simulink library "PEACDC01MSEREF"  (R2014b)
settings: Solver=ode45  StartTime=0.0  StopTime=10.0  RelTol=1e-3
undefined symbols (not defined in the file): errordlg
libraries: simulink x6
settings Model: Creator=vda2sh  LastModifiedBy=vda2sh
settings OptimizationCC: UseDivisionForNetSlopeComputation=off  SimCompilerOptimization=off
settings DebuggingCC: FrameProcessingCompatibilityMsg=error  AllowSymbolicDim=off
settings RTWCC: RTWCompilerOptimization=off
settings ConfigComp: CovMetricSettings=dw  CovHtmlReporting=on  CovSaveCumulativeToWorkspaceVar=on  CovSaveSingleToWorkspaceVar=on  CovModelRefEnable=Off  CovExternalEMLEnable=off  CovSFcnEnable=off

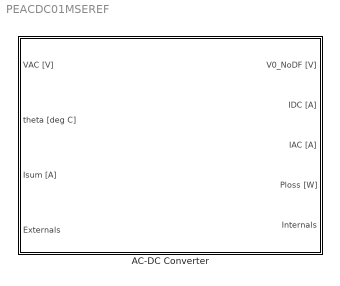
== system PEACDC01MSEREF ==
  "AC-DC Converter " : Subsystem  Tag=PEACDC01MSEREF  RequirementInfo="{}  %GIDa_5dfe5db4_0575_4ff1_ab59_fb674d557647"  mask(PEACDC01MSEREF){VD20=0.7, RD20=1e-3, alphaVD=0.0, alphaRD=0.0}
      mask prompts: VD20 "Diode forward voltage at 20°C [V]"; RD20 "Diode on resistance at 20°C [Ohm]"; alphaVD "Thermal coefficient of diode forward voltage [1/K]"; alphaRD "Thermal coefficient of diode on resistance [1/K]"
      mask help:
      | PEACDC01MSEREF - AC-DC converter
      |
      | This is a model of an AC-DC converter. It represents a full-wave rectifier using 4 diodes.
      settings: AttributesFormatString=<%<Tag>>
      mask Help: eval('show_docs_mseref_powerelectronics(''PEACDC01MSEREF'')')
      mask Display:
      | image(imread('PEACDC01MSEREF.jpg'),[0.16, 0.15, 0.73, 0.7]);
      | port_label('input',1,'VAC [V]')
      | port_label('input',2,'theta [°C]')
      | port_label('input',3,'Isum [A]')
      | port_label('input',4,'Externals')
      | port_label('output',1,'V0_NoDF [V]')
      | port_label('output',2,'IDC [A]')
      | port_label('output',3,'IAC [A]')
      | port_label('output',4,'Ploss [W]')
      | port_label('output',5,'Internals')

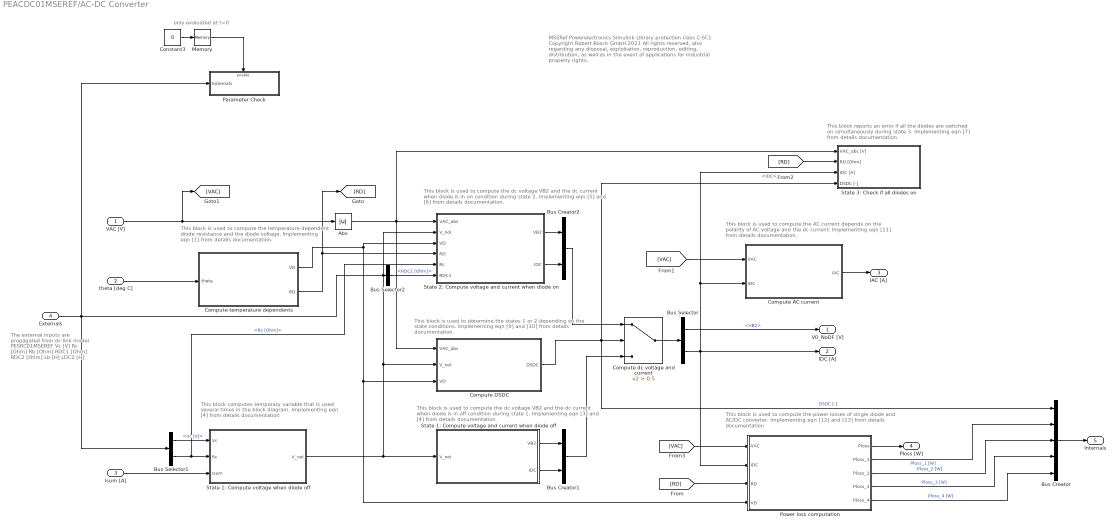
== system PEACDC01MSEREF/AC-DC Converter  ==
  note: The external inputs are
      | propagated from dc-link
      | model PESRC01MSEREF
      |
      | Vc [V]
      | Rc [Ohm]
      | Rb [Ohm]
      | RDC1 [Ohm]
      | RDC2 [Ohm]
      | Lb [H]
      | LDC2 [H]
  note: This block is used to compute the power losses of single diode
      | and AC/DC converter.
      | Implementing eqn [12] and [13] from details documentation
  note: This block is used to compute the AC current
      | depends on the polarity of AC voltage and the dc current.
      | Implementing eqn [11] from details documentation.
  note: This block reports an error if all the diodes
      | are switched on simultaneously during state 3.
      | Implementing eqn [7] from details documentation
  note: This block  computes temporary variable that is
      | used several times in the block diagram.
      | Implementing eqn [4] from details documentation
  note: This block is used to compute the dc voltage VB2
      |  and the dc current when diode is in off condition during state 1.
      | Implementing eqn [3] and [4] from details documentation
  note: This block is used to compute the dc voltage VB2
      |  and the dc current when diode is in on condition during state 2.
      | Implementing eqn [5] and [6] from details documentation.
  note: This block is used to compute
      | the temperature dependent diode resistance
      | and the diode voltage.
      | Implementing eqn [1] from details documentation.
  note: only evaluated at t=0
  note: This block is used to determine the states 1 or 2 depending
      | on the state conditions.
      | Implementing eqn [9] and [10] from details documentation.
  note: MSERef Powerelectronics Simulink Library
      | protection class C-SC1
      |
      | Copyright Robert Bosch GmbH 2021
      |
      | All rights reserved, also regarding any disposal, exploitation,
      | reproduction, editing, distribution, as well as in the event of
      | applications for industrial property rights.
  VAC [V] : Inport
  theta [deg C] : Inport  Port=2
  Isum [A] : Inport  Port=3
  Externals : Inport  Port=4
  Abs : Abs
  Bus Creator : BusCreator  Inputs=5
  Bus Creator1 : BusCreator  Inputs=2
  Bus Creator2 : BusCreator  Inputs=2
  Bus Selector : BusSelector  OutputSignals=VB2,IDC
  Bus Selector1 : BusSelector  OutputSignals=Vc [V],Rc [Ohm]
  Bus Selector2 : BusSelector  OutputSignals=RDC1 [Ohm]
  Compute AC current : MATLAB Function  TreatAsAtomicUnit=on
  Compute DSDC : MATLAB Function  TreatAsAtomicUnit=on
  Compute dc voltage and current : Switch  Criteria=u2 > Threshold  Threshold=0.5
  Compute temperature dependents : MATLAB Function  TreatAsAtomicUnit=on
  Constant3 : Constant  Value=0
  Memory : Memory  X0=1
  Parameter Check : Subsystem  TreatAsAtomicUnit=on
  Power loss computation : MATLAB Function  TreatAsAtomicUnit=on
  State 1: Compute voltage and current when diode off : MATLAB Function  TreatAsAtomicUnit=on
  State 1: Compute voltage when diode off : MATLAB Function  TreatAsAtomicUnit=on
  State 2: Compute voltage and current when diode on : MATLAB Function  TreatAsAtomicUnit=on
  State 3: Check if all diodes on : Subsystem
  V0_NoDF [V] : Outport
  IDC [A] : Outport  Port=2
  IAC [A] : Outport  Port=3
  Ploss [W] : Outport  Port=4
  Internals : Outport  Port=5
  wires:
  Bus Selector2/1 -> State 2: Compute voltage and current when diode on/6(RDC1)  "<RDC1 [Ohm]>"
  Bus Selector1/1 -> State 1: Compute voltage when diode off/1(Vc)  "<Vc [V]>"
  VAC [V]/1 -> Abs/1, [VAC]
  State 1: Compute voltage and current when diode off/1(VB2) -> Bus Creator1/1
  Bus Selector/1 -> V0_NoDF [V]/1  "<VB2>"
  Bus Selector1/2 -> State 2: Compute voltage and current when diode on/5(Rc), State 1: Compute voltage when diode off/2(Rc)  "<Rc [Ohm]>"
  Isum [A]/1 -> State 1: Compute voltage when diode off/3(Isum)
  Bus Selector/2 -> Power loss computation/2(IDC), State 3: Check if all diodes on/3(IDC [A]), Compute AC current/2(IDC), IDC [A]/1  "<IDC>"
  Bus Creator1/1 -> Compute dc voltage and current/3
  Externals/1 -> Bus Selector1/1, Bus Selector2/1, Parameter Check/1(Externals)
  State 2: Compute voltage and current when diode on/2(IDC) -> Bus Creator2/2
  State 1: Compute voltage and current when diode off/2(IDC) -> Bus Creator1/2
  State 1: Compute voltage when diode off/1(V_noI) -> State 2: Compute voltage and current when diode on/2(V_noI), Compute DSDC/2(V_noI), State 1: Compute voltage and current when diode off/1(V_noI)
  Compute temperature dependents/1(VD) -> Power loss computation/4(VD), Compute DSDC/3(VD), State 2: Compute voltage and current when diode on/3(VD)
  State 2: Compute voltage and current when diode on/1(VB2) -> Bus Creator2/1
  Compute AC current/1(IAC) -> IAC [A]/1
  Bus Creator2/1 -> Compute dc voltage and current/1
  Compute dc voltage and current/1 -> Bus Selector/1
  Compute temperature dependents/2(RD) -> State 2: Compute voltage and current when diode on/4(RD), [RD]
  [RD] -> Power loss computation/3(RD)
  Power loss computation/1(Ploss) -> Ploss [W]/1
  Abs/1 -> State 3: Check if all diodes on/1(VAC_abs [V]), Compute DSDC/1(VAC_abs), State 2: Compute voltage and current when diode on/1(VAC_abs)
  Constant3/1 -> Memory/1
  theta [deg C]/1 -> Compute temperature dependents/1(theta)
  Memory/1 -> Parameter Check/Enable
  Bus Creator/1 -> Internals/1
  [VAC] -> Power loss computation/1(VAC)
  [VAC] -> Compute AC current/1(VAC)
  Compute DSDC/1(DSDC) -> State 3: Check if all diodes on/4(DSDC [-]), Bus Creator/1, Compute dc voltage and current/2  "DSDC [-]"
  Power loss computation/4(Ploss_3) -> Bus Creator/4  "Ploss_3 [W]"
  Power loss computation/5(Ploss_4) -> Bus Creator/5  "Ploss_4 [W]"
  Power loss computation/3(Ploss_2) -> Bus Creator/3  "Ploss_2 [W]"
  Power loss computation/2(Ploss_1) -> Bus Creator/2  "Ploss_1 [W]"
  [RD] -> State 3: Check if all diodes on/2(RD [Ohm])

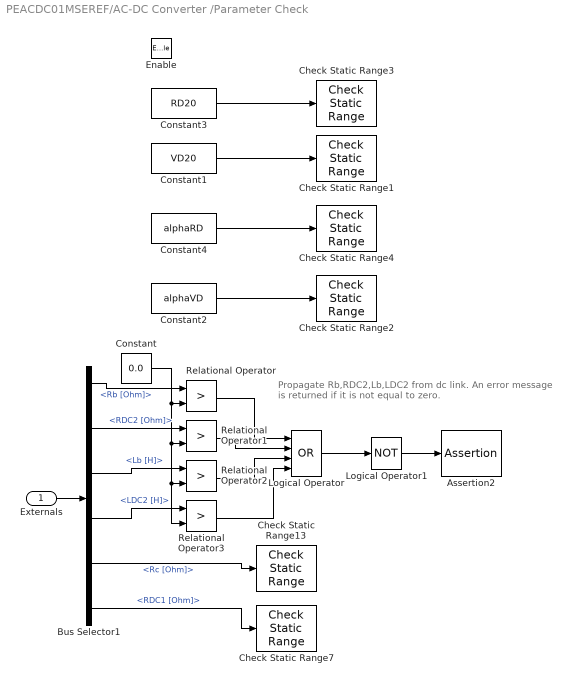
== system PEACDC01MSEREF/AC-DC Converter /Parameter Check ==
  note: Propagate Rb,RDC2,Lb,LDC2 from dc link. An error message is returned if it is not equal to zero.
  Externals : Inport
  Enable : EnablePort
  Assertion2 : Assertion  AssertionFailFcn=errordlg('For proper coupling between ACDC and DC link following variables Rb, RDC2, Lb, LDC2 must be set to zero. It considers only wire harness ohmic resistance effects')
  Bus Selector1 : BusSelector  OutputSignals=Rb [Ohm],RDC2 [Ohm],Lb [H],LDC2 [H],Rc [Ohm],RDC1 [Ohm]
  Check Static Range{1..4,7,13} (6 alike) : simulink/Model Verification/Check  Static Range  Description=0 <= u <= 100  max=100  max_included=on  min=0  min_included=on  enabled=on  stopWhenAssertionFail=on  export=off  icon=graphic
  Constant : Constant  Value=0.0
  Constant1 : Constant  Value=VD20
  Constant2 : Constant  Value=alphaVD
  Constant3 : Constant  Value=RD20
  Constant4 : Constant  Value=alphaRD
  Logical Operator : Logic  Operator=OR  Inputs=4  AllPortsSameDT=off  OutDataTypeStr=boolean
  Logical Operator1 : Logic  Operator=NOT  AllPortsSameDT=off  OutDataTypeStr=boolean
  Relational Operator{,1..3} (4 alike) : RelationalOperator  Operator=>  OutDataTypeStr=boolean
  wires:
  Bus Selector1/5 -> Check Static Range13/1  "<Rc [Ohm]>"
  Logical Operator1/1 -> Assertion2/1
  Logical Operator/1 -> Logical Operator1/1
  Relational Operator3/1 -> Logical Operator/4
  Relational Operator2/1 -> Logical Operator/3
  Relational Operator1/1 -> Logical Operator/2
  Relational Operator/1 -> Logical Operator/1
  Constant/1 -> Relational Operator3/2, Relational Operator2/2, Relational Operator1/2, Relational Operator/2
  Bus Selector1/4 -> Relational Operator3/1  "<LDC2 [H]>"
  Bus Selector1/3 -> Relational Operator2/1  "<Lb [H]>"
  Bus Selector1/2 -> Relational Operator1/1  "<RDC2 [Ohm]>"
  Bus Selector1/1 -> Relational Operator/1  "<Rb [Ohm]>"
  Externals/1 -> Bus Selector1/1
  Constant3/1 -> Check Static Range3/1
  Constant4/1 -> Check Static Range4/1
  Constant1/1 -> Check Static Range1/1
  Constant2/1 -> Check Static Range2/1
  Bus Selector1/6 -> Check Static Range7/1  "<RDC1 [Ohm]>"

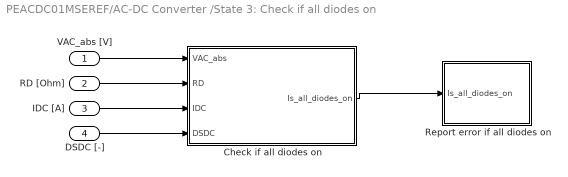
== system PEACDC01MSEREF/AC-DC Converter /State 3: Check if all diodes on ==
  VAC_abs [V] : Inport
  RD [Ohm] : Inport  Port=2
  IDC [A] : Inport  Port=3
  DSDC [-] : Inport  Port=4
  " Check if all diodes on" : MATLAB Function  TreatAsAtomicUnit=on
  "Report error if all diodes on " : Subsystem
  wires:
  RD [Ohm]/1 -> " Check if all diodes on"/2(RD)
  " Check if all diodes on"/1(Is_all_diodes_on) -> "Report error if all diodes on "/1(Is_all_diodes_on)
  IDC [A]/1 -> " Check if all diodes on"/3(IDC)
  VAC_abs [V]/1 -> " Check if all diodes on"/1(VAC_abs)
  DSDC [-]/1 -> " Check if all diodes on"/4(DSDC)

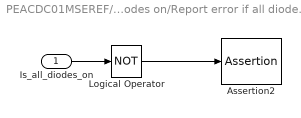
== system PEACDC01MSEREF/AC-DC Converter /State 3: Check if all diodes on/Report error if all diodes on  ==
  Is_all_diodes_on : Inport
  Assertion2 : Assertion  AssertionFailFcn=errordlg('All diodes are switched on simultaneously. Either Isum current is too high or Vc voltage is too low.')
  Logical Operator : Logic  Operator=NOT  AllPortsSameDT=off  OutDataTypeStr=boolean
  wires:
  Logical Operator/1 -> Assertion2/1
  Is_all_diodes_on/1 -> Logical Operator/1

== matlab function PEACDC01MSEREF/AC-DC Converter /Compute AC current ==
  data: IAC output; VAC input; IDC input
function IAC  = fcn(VAC,IDC)
%  This function is used to compute the AC current 
%  depends on the polarity of AC voltage and the dc current.
%
%  MSERef Powerelectronics Simulink Library 
%  protection class C-SC1
%
%  Copyright Robert Bosch GmbH 2021
%
%  All rights reserved, also regarding any disposal, exploitation,
%  reproduction, editing, distribution, as well as in the event of
%  applications for industrial property rights.

  
%#codegen

%Output AC current Implementing Eqn [11] 
if VAC >= 0.0
    IAC = IDC;
else
    IAC = -IDC;    
end

== matlab function PEACDC01MSEREF/AC-DC Converter /Compute DSDC ==
  data: DSDC output; VAC_abs input; V_noI input; VD input
function DSDC  = fcn(VAC_abs,V_noI,VD)
% This function is used to determine the state 1 or 2 depending
% on the state conditions.
%
%  MSERef Powerelectronics Simulink Library 
%  protection class C-SC1
%
%  Copyright Robert Bosch GmbH 2021
%
%  All rights reserved, also regarding any disposal, exploitation,
%  reproduction, editing, distribution, as well as in the event of
%  applications for industrial property rights.

  
%#codegen

%State 1: Implementing Eqn [9]
if (VAC_abs - V_noI <= 2*VD) 
    %Diodes OFF
    DSDC = 0;
else  
    %State 2: Implementing Eqn [10]
    %Diodes ON
    DSDC = 1;     
end

== matlab function PEACDC01MSEREF/AC-DC Converter /Compute temperature dependents ==
  data: VD output; theta input; RD output; VD20 parameter; RD20 parameter; alphaVD parameter; alphaRD parameter
function [VD, RD] = fcn(theta, VD20, RD20, alphaVD, alphaRD)
% This function is used to compute the temperature dependent diode
% resistance and voltage
%
%  MSERef Powerelectronics Simulink Library 
%  protection class C-SC1
%
%  Copyright Robert Bosch GmbH 2021
%
%  All rights reserved, also regarding any disposal, exploitation,
%  reproduction, editing, distribution, as well as in the event of
%  applications for industrial property rights.

  
%#codegen

%Implementing Eqn [1]
%Calculation of temperature dependent diode forward voltage 
VD = VD20 *(1 + alphaVD *(theta - 20));

%Calculation of temperature dependent diode resistance 
RD = RD20 *(1 + alphaRD *(theta - 20));

== matlab function PEACDC01MSEREF/AC-DC Converter /Power loss computation ==
  data: Ploss output; Ploss_1 output; Ploss_2 output; Ploss_3 output; Ploss_4 output; VAC input; IDC input; RD input; VD input
function [Ploss,Ploss_1,Ploss_2,Ploss_3,Ploss_4] = fcn(VAC,IDC, RD, VD)
%  This function is used to compute the power losses of single diode
%  and AC/DC converter.
%
%  MSERef Powerelectronics Simulink Library 
%  protection class C-SC1
%
%  Copyright Robert Bosch GmbH 2021
%
%  All rights reserved, also regarding any disposal, exploitation,
%  reproduction, editing, distribution, as well as in the event of
%  applications for industrial property rights.

  
%#codegen

%Conducting power loss of AC/DC converter: Implementing Eqn [13]
Ploss = 2*(VD*IDC + RD * IDC^2);  

Ploss_1 = 0.0;
Ploss_2 = 0.0;
Ploss_3 = 0.0;
Ploss_4 = 0.0;

%Conducting power loss of each diode: Implementing Eqn [12]
if VAC >= 0    
    Ploss_1 = VD*IDC + RD * IDC^2;
    Ploss_4 = VD*IDC + RD * IDC^2;
else
    Ploss_2 = VD*IDC + RD * IDC^2;
    Ploss_3 = VD*IDC + RD * IDC^2;
end

== matlab function PEACDC01MSEREF/AC-DC Converter /State 1: Compute voltage and current when diode off ==
  data: VB2 output; V_noI input; IDC output
function [VB2,IDC]  = fcn(V_noI)
% This function is used to compute dc voltage VB2
% and the dc current when diode is in off condition during state 1.
%
%  MSERef Powerelectronics Simulink Library 
%  protection class C-SC1
%
%  Copyright Robert Bosch GmbH 2021
%
%  All rights reserved, also regarding any disposal, exploitation,
%  reproduction, editing, distribution, as well as in the event of
%  applications for industrial property rights.

  
%#codegen


%Output DC voltage: Implementing Eqn [4]
VB2  = V_noI;

%Output DC current: Implementing Eqn [3]
IDC  = 0.0; 

end

== matlab function PEACDC01MSEREF/AC-DC Converter /State 1: Compute voltage when diode off ==
  data: V_noI output; Vc input; Rc input; Isum input
function V_noI  = fcn(Vc,Rc,Isum)
%  This function  computes temporary variable that is 
%  used several times in the block diagram.
%
%  MSERef Powerelectronics Simulink Library 
%  protection class C-SC1
%
%  Copyright Robert Bosch GmbH 2021
%
%  All rights reserved, also regarding any disposal, exploitation,
%  reproduction, editing, distribution, as well as in the event of
%  applications for industrial property rights.

  
%#codegen

%Output dc voltage when no current in the diode: Implementing Eqn [4]
V_noI = Vc - Rc*Isum;

end

== matlab function PEACDC01MSEREF/AC-DC Converter /State 2: Compute voltage and current when diode on ==
  data: VB2 output; VAC_abs input; V_noI input; VD input; IDC output; RD input; Rc input; RDC1 input
function [VB2,IDC]  = fcn(VAC_abs,V_noI,VD,RD,Rc,RDC1)
% This function is used to compute dc voltage VB2
% and the dc current when diode is in on condition during state 2.
%
%  MSERef Powerelectronics Simulink Library 
%  protection class C-SC1
%
%  Copyright Robert Bosch GmbH 2021
%
%  All rights reserved, also regarding any disposal, exploitation,
%  reproduction, editing, distribution, as well as in the event of
%  applications for industrial property rights.

  
%#codegen

%Output DC current: Implementing Eqn [5] 
IDC = (VAC_abs - 2 * VD - V_noI )/(2*RD + RDC1 + Rc);

%Output DC voltage: Implementing Eqn [6]
VB2 = VAC_abs - 2 * (VD + RD * IDC);
end

== matlab function PEACDC01MSEREF/AC-DC Converter /State 3: Check if all diodes on/ Check if all diodes on ==
  data: Is_all_diodes_on output; VAC_abs input; RD input; IDC input; DSDC input
function Is_all_diodes_on  = fcn(VAC_abs,RD,IDC,DSDC)
%  This function reports an error if all the diodes 
%  are switched on simultaneously during state 3.
%
%  MSERef Powerelectronics Simulink Library 
%  protection class C-SC1
%
%  Copyright Robert Bosch GmbH 2021
%
%  All rights reserved, also regarding any disposal, exploitation,
%  reproduction, editing, distribution, as well as in the event of
%  applications for industrial property rights.

  
%#codegen

Is_all_diodes_on = 0;

if DSDC > 0.5
    %State 3: Implementing Eqn [7]
    if VAC_abs < IDC*RD
        Is_all_diodes_on = 1;
    else
        Is_all_diodes_on = 0;
    end
end
